simulink model "lqg_controller"  (R2024b)
settings: Solver=VariableStepAuto  StartTime=0.0  StopTime=80  RelTol=1e-3
values from neighbouring files (symbols this model uses):
  An = double(subs(Af,{M,m1,m2,l1,l2,g},{1000,100,100,20,10,9.81}))    [PartD_LQRController.m]    (also in PartF_luenberger_observers.m; PartG_LQG_controller.m)
  Bn = double(subs(Bf,{M,m1,m2,l1,l2,g},{1000,100,100,20,10,9.81}))    [PartD_LQRController.m]    (also in PartF_luenberger_observers.m; PartG_LQG_controller.m)
  C = eye(6,6)    [PartB_linearization.m]    (also in PartC_contollability_condition.m; PartD_LQRController.m; PartG_LQG_controller.m = [  0 0 0 0 0 0)
  D = [0;0;0;0;0;0]    [PartB_linearization.m]    (also in PartC_contollability_condition.m; PartD_LQRController.m; PartE_observbliltiy_check.m; PartF_luenberger_observers.m)
  Rn = 0.1    [PartG_LQG_controller.m]
  x0 = [0;0;0;0;0.1;-0.1]    [PartB_linearization.m]    (also in PartC_contollability_condition.m = [0;0;0;0;0;0]; PartD_LQRController.m = [0;0;0;5;0;0]; PartE_observbliltiy_check.m = [0;0;0;0;0;0]; PartF_luenberger_observers.m = [0;0;0;0;0;0])
undefined symbols (not defined in the file or in its folder): Continuous, K, Time
libraries: ctrlSharedLib x1

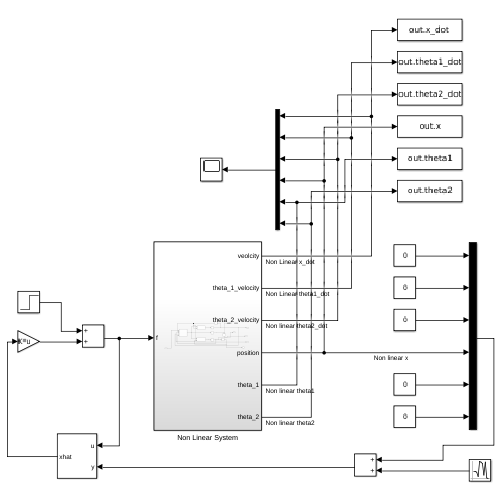
[thumbnail: Simulink's stored preview of the top-level diagram]
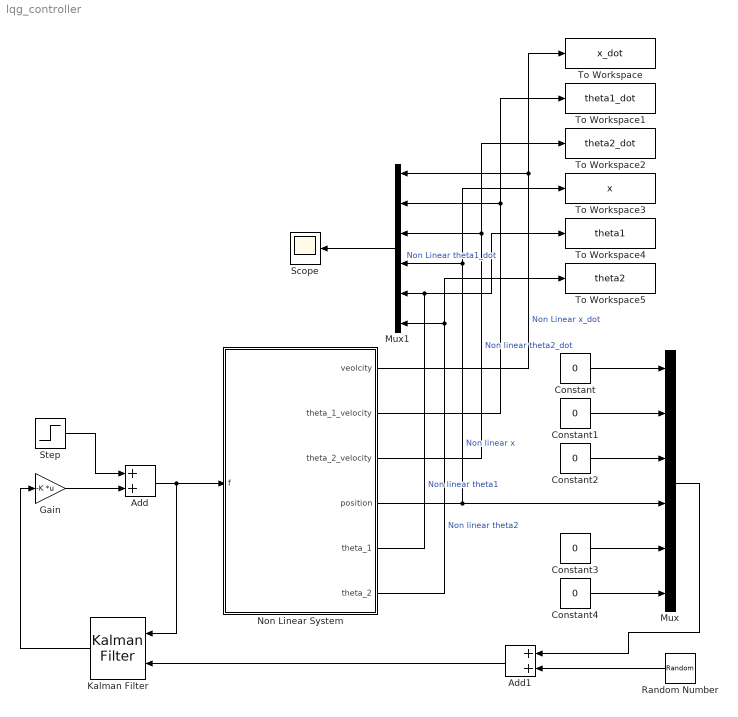
== system lqg_controller ==
  Add : Sum
  Add1 : Sum
  Constant{,1..4} (5 alike) : Constant  Value=0
  Gain : Gain  Gain=-K  Multiplication=Matrix(K*u)
  Kalman Filter : ctrlSharedLib/Kalman Filter  TimeDomain=Continuous-Time  UseCurrentEstimator=on  ModelSource=Individual A, B, C, D matrices  ModelSourceVariable=ss(0.95,1,1,0,1)  A=An  B=Bn  C=C  D=D  NumberOfStates=1  NumberOfInputs=1  NumberOfOutputs=1  InitialEstimateSource=Dialog  X0=x0  P0=10  UseK=off  UseGH=off  NumberOfProcessNoiseInputs=1  G=1  TimeInvariantG=on  H=0  TimeInvariantH=on  Q=Qn  TimeInvariantQ=on  R=Rn  TimeInvariantR=on  N=0  TimeInvariantN=on  AddInputPort=on  AddEnablePort=off  OutputEstimatedY=off  OutputP=off  Ts=-1
  Mux : Mux  Inputs=6
  Mux1 : Mux  Inputs=6
  Non Linear System : Subsystem
  Random Number : RandomNumber  Variance=Rn  SampleTime=0.1
  Scope : Scope
  Step : Step  After=1000  SampleTime=0
  To Workspace : ToWorkspace  VariableName=x_dot  SaveFormat=Timeseries  SampleTime=-1
  To Workspace1 : ToWorkspace  VariableName=theta1_dot  SaveFormat=Timeseries  SampleTime=-1
  To Workspace2 : ToWorkspace  VariableName=theta2_dot  SaveFormat=Timeseries  SampleTime=-1
  To Workspace3 : ToWorkspace  VariableName=x  SaveFormat=Timeseries  SampleTime=-1
  To Workspace4 : ToWorkspace  VariableName=theta1  SaveFormat=Timeseries  SampleTime=-1
  To Workspace5 : ToWorkspace  VariableName=theta2  SaveFormat=Timeseries  SampleTime=-1
  wires:
  Non Linear System/4(position) -> To Workspace3/1, Mux1/4, Mux/4  "Non linear x"
  Gain/1 -> Add/2
  Add/1 -> Kalman Filter/1, Non Linear System/1(f)
  Step/1 -> Add/1
  Constant4/1 -> Mux/6
  Constant3/1 -> Mux/5
  Constant2/1 -> Mux/3
  Constant1/1 -> Mux/2
  Constant/1 -> Mux/1
  Non Linear System/1(veolcity) -> To Workspace/1, Mux1/1  "Non Linear x_dot"
  Non Linear System/6(theta_2) -> To Workspace5/1, Mux1/6  "Non linear theta2"
  Non Linear System/5(theta_1) -> Mux1/5, To Workspace4/1  "Non linear theta1"
  Non Linear System/3(theta_2_velocity) -> To Workspace2/1, Mux1/3  "Non linear theta2_dot"
  Non Linear System/2(theta_1_velocity) -> Mux1/2, To Workspace1/1  "Non Linear theta1_dot"
  Mux1/1 -> Scope/1
  Kalman Filter/1 -> Gain/1
  Add1/1 -> Kalman Filter/2
  Random Number/1 -> Add1/2
  Mux/1 -> Add1/1

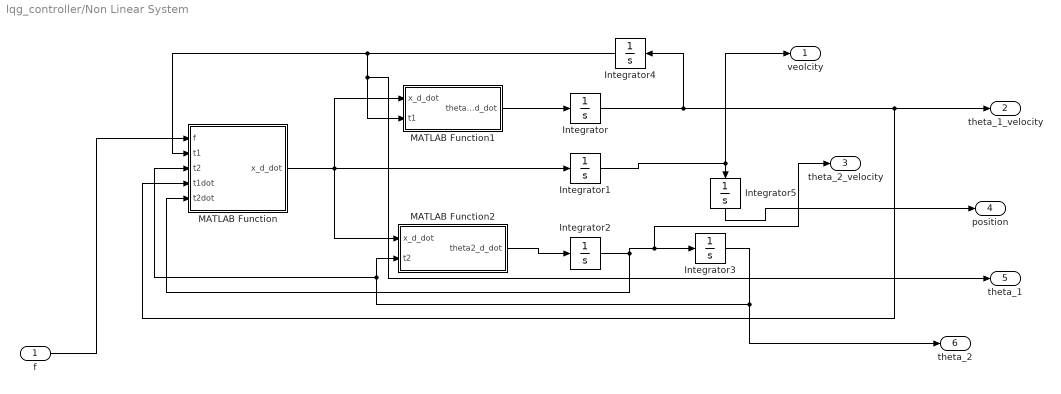
== system lqg_controller/Non Linear System ==
  f : Inport
  Integrator : Integrator  InitialCondition=x0(2)
  Integrator1 : Integrator  InitialCondition=x0(1)
  Integrator2 : Integrator  InitialCondition=x0(3)
  Integrator3 : Integrator  InitialCondition=x0(6)
  Integrator4 : Integrator  InitialCondition=x0(5)
  Integrator5 : Integrator  InitialCondition=x0(4)
  MATLAB Function : MATLAB Function  TreatAsAtomicUnit=on
  MATLAB Function1 : MATLAB Function  TreatAsAtomicUnit=on
  MATLAB Function2 : MATLAB Function  TreatAsAtomicUnit=on
  veolcity : Outport
  theta_1_velocity : Outport  Port=2
  theta_2_velocity : Outport  Port=3
  position : Outport  Port=4
  theta_1 : Outport  Port=5
  theta_2 : Outport  Port=6
  wires:
  f/1 -> MATLAB Function/1(f)
  MATLAB Function2/1(theta2_d_dot) -> Integrator2/1
  MATLAB Function1/1(theta1_d_dot) -> Integrator/1
  Integrator5/1 -> position/1
  Integrator1/1 -> veolcity/1, Integrator5/1
  Integrator2/1 -> theta_2_velocity/1, Integrator3/1, MATLAB Function/5(t2dot)
  Integrator/1 -> Integrator4/1, theta_1_velocity/1, MATLAB Function/4(t1dot)
  Integrator4/1 -> theta_1/1, MATLAB Function1/2(t1), MATLAB Function/2(t1)
  MATLAB Function/1(x_d_dot) -> Integrator1/1, MATLAB Function1/1(x_d_dot), MATLAB Function2/1(x_d_dot)
  Integrator3/1 -> theta_2/1, MATLAB Function/3(t2), MATLAB Function2/2(t2)

== matlab function lqg_controller/Non Linear System/MATLAB Function1 ==
  data: x_d_dot input; theta1_d_dot output; t1 input
function theta1_d_dot = fcn(x_d_dot,t1)

l1 = 20;
theta1_d_dot = (cos(t1)*x_d_dot - 9.81*sin(t1))/l1;

== matlab function lqg_controller/Non Linear System/MATLAB Function ==
  settings: updateMethod=DISCRETE
  data: f input; x_d_dot output; t1 input; t2 input; t1dot input; t2dot input
function x_d_dot = fcn(f,t1,t2,t1dot,t2dot)

M = 1000;
m1 = 100;
m2 = 100;
g = 9.81;
l1 = 20;
l2 = 10;
Q = 0.05;
noise = sqrt(Q) * randn;

x_d_dot = noise + (f - m1*l1*sin(t1)*t1dot^2 -m2*l2*sin(t2)*t2dot^2 -m1*g*sin(t1)*cos(t1) - m2*g*sin(t2)*cos(t2))/(M + m1*(sin(t1))^2 + m2*(sin(t2))^2);

== matlab function lqg_controller/Non Linear System/MATLAB Function2 ==
  data: x_d_dot input; theta2_d_dot output; t2 input
function theta2_d_dot = fcn(x_d_dot,t2)

l2 = 10;
theta2_d_dot = (cos(t2)*x_d_dot - 9.81*sin(t2))/l2;
